simulink model "gm_Encoder_Zynq_vnl"  (R2018a)
settings: Solver=ode3  StartTime=0.0  StopTime=SimulationsDauer  RelTol=1e-3  EnableMultiTasking=on
undefined symbols (not defined in the file or in its folder): DiscIntNeverNeededParam, f_ISR, IncPerTurn, n_max, OverSamplingFactor, OverSamplingFactorInverse, Periode, Phase_Delay_A, Phase_Delay_B, PolePair, T_mech, TestDrehzahl_rpm
libraries: simulink x18, hdlsllib x2, dspsigops x2, dspswit3 x2, powerlib_meascontrol x2, hdlmdlgenlib x1, simulink_extras x1, powerlib x1
(part 1 of 3)
settings Model: Creator=Wendel_ELSYS  LastModifiedBy=Wendel
settings DataIOCC: LimitDataPoints=on  SaveFormat=Array
settings OptimizationCC: BlockReduction=off  ConditionallyExecuteInputs=off  DefaultParameterBehavior=Inlined  LifeSpan=inf
settings DebuggingCC: AlgebraicLoopMsg=error  InheritedTsInSrcMsg=none  ParameterOverflowMsg=none  SFUnexpectedBacktrackingDiag=warning  SFNoUnconditionalDefaultTransitionDiag=warning  SFExecutionAtInitializationDiag=none
settings HardwareCC: ProdBitPerPointer=32  ProdBitPerSizeT=32  ProdBitPerPtrDiffT=32  ProdLargestAtomicFloat=None  ProdIntDivRoundTo=Undefined  ProdEndianess=Unspecified  ProdWordSize=32  ProdHWDeviceType=ASIC/FPGA->ASIC/FPGA  ProdEqTarget=off
settings ModelReferenceCC: PropagateSignalLabelsOutOfModel=off
settings CodeAppCC: StateflowObjectComments=on
settings GRTTargetCC: TargetLangStandard=C89/C90 (ANSI)  GeneratePreprocessorConditionals=Disable all
settings ConfigComp: CovMetricSettings=dw  CovHtmlReporting=on  CovSaveCumulativeToWorkspaceVar=on  CovSaveSingleToWorkspaceVar=on  CovExternalEMLEnable=off
settings SimscapeCC: SimscapeNormalizeSystem=off

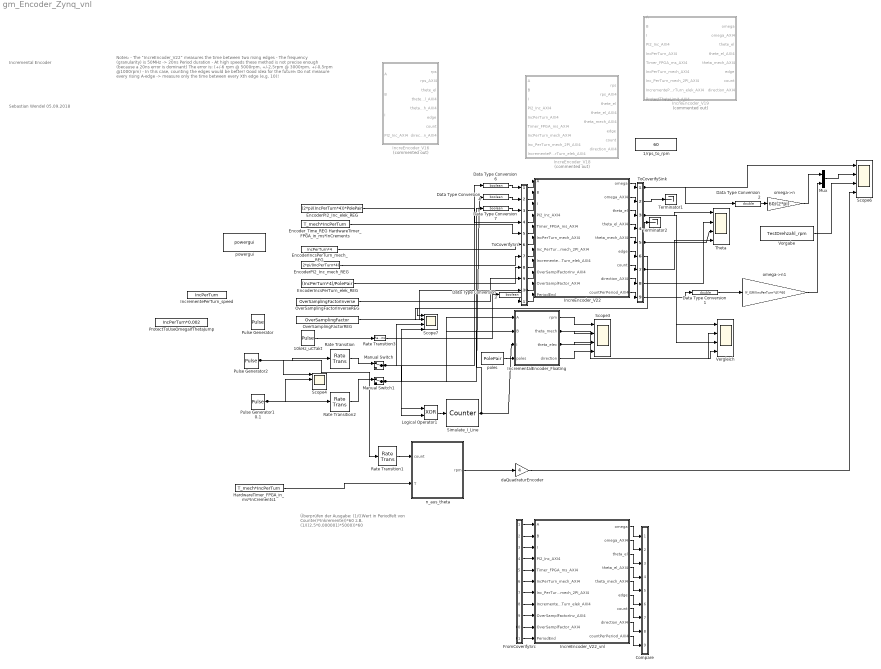
== system gm_Encoder_Zynq_vnl ==
  note: Überprüfen der Ausgabe:
      | (1/((Wert in Periodfelt von Counter)*Inkremente))*60
      | z.B. (1/((2.5*0.000001)*5000))*60
  note: Sebastian Wendel
      | 05.09.2018
  note: Notes:
      | - The "IncreEncoder_V22" measures the time between two rising edges
      | - The frequency (granularity) is 50MHz -> 20ns Period duration
      | - At high speeds these method is not precise enough (because a 20ns error is dominant)
      | The error is: (+/-6 rpm @ 5000rpm, +/-2,5rpm @ 3000rpm, +/-0,5rpm @1000rpm)
      | - In this case, counting the edges would be better!
      |
      | Good idea for the future: Do not measure every rising A-edge
      | -> measure only the time between every Xth edge (e.g. 10)!
  note: Incremental Encoder
  1/rps_to_rpm : Constant  Value=60  OutDataTypeStr=double  SampleTime=T_mech
  10kHz_uCTakt : DiscretePulseGenerator  PulseType=Time based  Period=0.000100  PulseWidth=0.0002  SampleTime=T_mech  VectorParams1D=off
  Compare : Subsystem
      mask Display: disp('')
  Data Type Conversion1 : DataTypeConversion  OutDataTypeStr=double
  Data Type Conversion2 : DataTypeConversion  OutDataTypeStr=double
  Data Type Conversion{3..4,6..7} (4 alike) : DataTypeConversion  OutDataTypeStr=boolean
  "EncoderIncsPerTurn_elek_REG " : Constant  Value=(IncPerTurn*4)/PolePair  OutDataTypeStr=fixdt(0,16,0)  SampleTime=T_mech
  EncoderIncsPerTurn_mech_REG : Constant  Value=IncPerTurn*4  OutDataTypeStr=fixdt(0,16,0)  SampleTime=T_mech
  EncoderPI2_Inc_elek_REG : Constant  Value=(2*pi/(IncPerTurn*4))*PolePair  OutDataTypeStr=fixdt(0,24,24)  SampleTime=T_mech
  EncoderPI2_Inc_mech_REG : Constant  Value=2*pi/(IncPerTurn*4)  OutDataTypeStr=fixdt(0,24,24)  SampleTime=T_mech
  Encoder_Time_REG HardwareTimer_FPGA_in_ms*InCrements : Constant  Value=T_mech*IncPerTurn  OutDataTypeStr=fixdt(0,32,26)  SampleTime=T_mech
  FromCoverifySrc : Subsystem
      mask Display: disp('')
  HardwareTimer_FPGA_in_ms*InCrements1 : Constant  Value=T_mech*IncPerTurn  OutDataTypeStr=double  SampleTime=T_mech
  IncreEncoder_V16 : Subsystem  Commented=on  TreatAsAtomicUnit=on
  IncreEncoder_V18 : Subsystem  Commented=on  TreatAsAtomicUnit=on
  IncreEncoder_V19 : Subsystem  Commented=on  TreatAsAtomicUnit=on
  IncreEncoder_V22 : Subsystem  TreatAsAtomicUnit=on
  IncreEncoder_V22_vnl : Subsystem  TreatAsAtomicUnit=on
  IncrementalEncoder_Floating : Subsystem
  IncrementePerTurn_speed : Constant  Value=IncPerTurn  OutDataTypeStr=fixdt(0,16,0)  SampleTime=T_mech
  Logical Operator1 : Logic  Operator=XOR  AllPortsSameDT=off  OutDataTypeStr=boolean
  Manual Switch : ManualSwitch
  Manual Switch1 : ManualSwitch
  Mux : Mux  Inputs=2
  OverSamplingFactorInverseREG : Constant  Value=OverSamplingFactorInverse  OutDataTypeStr=fixdt(0,16,15)  SampleTime=T_mech
  OverSamplingFactorREG : Constant  Value=OverSamplingFactor  OutDataTypeStr=fixdt(0,16,0)  SampleTime=T_mech
  ProtectToUseOmegaIfThetaJump : Constant  Value=IncPerTurn*0.002  OutDataTypeStr=uint16  SampleTime=T_mech
  Pulse Generator : DiscretePulseGenerator  PulseType=Time based  Period=0.01  PulseWidth=50  PhaseDelay=0.00000125  SampleTime=T_mech  VectorParams1D=off
  Pulse Generator1 0.1 : DiscretePulseGenerator  PulseType=Time based  Period=Periode  PulseWidth=50  PhaseDelay=Phase_Delay_B  SampleTime=T_mech  VectorParams1D=off
  Pulse Generator2 : DiscretePulseGenerator  PulseType=Time based  Period=Periode  PulseWidth=50  PhaseDelay=Phase_Delay_A  SampleTime=T_mech  VectorParams1D=off
  Rate Transition{,1..3} (4 alike) : RateTransition  Deterministic=off  OutPortSampleTime=T_mech
  Scope{3..4,6..7} (4 alike) : Scope  NumInputPorts=4
  Simulate_I_Line : dspswit3/Counter  Direction=Up  CountEvent=Either edge  CounterSize=User defined  MaxCount=IncPerTurn*4  InitialCount=0  Output=Hit  HitValue=IncPerTurn*4  ResetInput=off  SamplesPerFrame=1  Ts=1  CntDtype=double  HitDtype=Boolean
  Terminator1 : Terminator
  Terminator2 : Terminator
  Theta : Scope  NumInputPorts=4
  ToCoverifySink : Subsystem
      mask Display: disp('')
  ToCoverifySrc : Subsystem
      mask Display: disp('')
  Vergleich : Scope  NumInputPorts=4
  Vorgabe : Constant  Value=TestDrehzahl_rpm
  "daQuadraturEncoder " : Gain  Gain=4
  n_aus_theta : Subsystem  TreatAsAtomicUnit=on
  omega->n : Gain  Gain=60/(2*pi)  OutDataTypeStr=double
  omega->n1 : Gain  Gain=(f_ISR/(IncPerTurn*4))*60  OutDataTypeStr=double
  poles : Constant  Value=PolePair  OutDataTypeStr=uint8  SampleTime=-1
  powergui : powerlib/powergui  Priority=1  SimulationMode=Discrete  SampleTime=T_mech  frequency=60  Iterations=50  frequencyindice=0  Pbase=100e6  ErrMax=1e-4  UnitsV=kV  UnitsW=MW  buscounter=0  FunctionMessages=off  echomessages=off  EnableUseOfTLC=off  CurrentSourceSwitches=off  DisableSnubberDevices=off  DisableRonSwitches=off  DisableVfSwitches=off  DisplayEquations=off  SolverType=Tustin  Interpol=off  ExternalGateDelay=off  methode=off  Ts=0  x0status=blocks  SPID=off  SwTol=0  HookPort=off  RestoreLinks=warning  ResistiveCurrentMeasurement=off  Frange=[0:2:500]  Ylog=off  Xlog=on  ShowGrid=off  save=off  variable=ZData  structure=0  ZoomFFT=on  StartTime=0.0  cycles=1  DisplayStyle=1  fundamental=60  FreqAxis=off  MaxFrequency=1000  frequencyindicesteady=1  RmsSteady=1  display=off
  wires:
  Pulse Generator1 0.1/1 -> Scope4/2, Rate Transition2/1
  Manual Switch1/1 -> Logical Operator1/2, Scope7/4, IncrementalEncoder_Floating/2(B), Data Type Conversion4/1
  Simulate_I_Line/1 -> IncrementalEncoder_Floating/3(I), Data Type Conversion7/1
  Logical Operator1/1 -> Simulate_I_Line/1
  Manual Switch/1 -> Scope7/3, Data Type Conversion6/1, IncrementalEncoder_Floating/1(A), Logical Operator1/1
  IncrementalEncoder_Floating/1(rpm) -> Scope3/1
  IncrementalEncoder_Floating/2(theta_mech) -> Vergleich/4, Scope3/2
  IncrementalEncoder_Floating/3(theta_elec) -> Vergleich/2, Scope3/3
  IncrementalEncoder_Floating/4(direction) -> Scope3/4
  poles/1 -> IncrementalEncoder_Floating/4(poles)
  omega->n/1 -> Mux/1
  Data Type Conversion2/1 -> omega->n/1
  HardwareTimer_FPGA_in_ms*InCrements1/1 -> n_aus_theta/2(T)
  Rate Transition1/1 -> n_aus_theta/1(count)
  n_aus_theta/1(rpm) -> "daQuadraturEncoder "/1
  Pulse Generator2/1 -> Rate Transition/1, Scope4/1, Rate Transition1/1
  "daQuadraturEncoder "/1 -> Scope6/4
  Vorgabe/1 -> Scope6/3
  Rate Transition2/1 -> Manual Switch1/1
  Rate Transition/1 -> Manual Switch/1
  10kHz_uCTakt/1 -> Rate Transition3/1
  Rate Transition3/1 -> Data Type Conversion3/1
  Data Type Conversion1/1 -> omega->n1/1
  Mux/1 -> Scope6/2
  omega->n1/1 -> Mux/2
  ToCoverifySrc/1(out1) -> IncreEncoder_V22/1(A)
  ToCoverifySrc/2(out2) -> IncreEncoder_V22/2(B)
  ToCoverifySrc/3(out3) -> IncreEncoder_V22/3(I)
  ToCoverifySrc/4(out4) -> IncreEncoder_V22/4(PI2_Inc_AXI4)
  ToCoverifySrc/5(out5) -> IncreEncoder_V22/5(Timer_FPGA_ms_AXI4)
  ToCoverifySrc/6(out6) -> IncreEncoder_V22/6(IncPerTurn_mech_AXI4)
  ToCoverifySrc/7(out7) -> IncreEncoder_V22/7(Inc_PerTurn_mech_2PI_AXI4)
  ToCoverifySrc/8(out8) -> IncreEncoder_V22/8(IncrementePerTurn_elek_AXI4)
  ToCoverifySrc/9(out9) -> IncreEncoder_V22/9(OverSamplFactorInv_AXI4)
  ToCoverifySrc/10(out10) -> IncreEncoder_V22/10(OverSamplFactor_AXI4)
  ToCoverifySrc/11(out11) -> IncreEncoder_V22/11(PeriodEnd)
  IncreEncoder_V22/1(omega) -> ToCoverifySink/1(in1)
  IncreEncoder_V22/2(omega_AXI4) -> ToCoverifySink/2(in2)
  IncreEncoder_V22/3(theta_el) -> ToCoverifySink/3(in3)
  IncreEncoder_V22/4(theta_el_AXI4) -> ToCoverifySink/4(in4)
  IncreEncoder_V22/5(theta_mech_AXI4) -> ToCoverifySink/5(in5)
  IncreEncoder_V22/6(edge) -> ToCoverifySink/6(in6)
  IncreEncoder_V22/7(count) -> ToCoverifySink/7(in7)
  IncreEncoder_V22/8(direction_AXI4) -> ToCoverifySink/8(in8)
  IncreEncoder_V22/9(countPerPeriod_AXI4) -> ToCoverifySink/9(in9)
  Data Type Conversion6/1 -> ToCoverifySrc/1(in1)
  Data Type Conversion4/1 -> ToCoverifySrc/2(in2)
  Data Type Conversion7/1 -> ToCoverifySrc/3(in3)
  EncoderPI2_Inc_elek_REG/1 -> ToCoverifySrc/4(in4)
  Encoder_Time_REG HardwareTimer_FPGA_in_ms*InCrements/1 -> ToCoverifySrc/5(in5)
  EncoderIncsPerTurn_mech_REG/1 -> ToCoverifySrc/6(in6)
  EncoderPI2_Inc_mech_REG/1 -> ToCoverifySrc/7(in7)
  "EncoderIncsPerTurn_elek_REG "/1 -> ToCoverifySrc/8(in8)
  OverSamplingFactorInverseREG/1 -> ToCoverifySrc/9(in9)
  OverSamplingFactorREG/1 -> ToCoverifySrc/10(in10)
  Data Type Conversion3/1 -> ToCoverifySrc/11(in11)
  ToCoverifySink/1(out1) -> Data Type Conversion2/1, Scope6/1
  ToCoverifySink/2(out2) -> Terminator1/1
  ToCoverifySink/3(out3) -> Vergleich/1, Theta/1
  ToCoverifySink/4(out4) -> Terminator2/1
  ToCoverifySink/5(out5) -> Theta/3, Vergleich/3
  ToCoverifySink/6(out6) -> Scope7/1
  ToCoverifySink/7(out7) -> Scope7/2, Theta/4
  ToCoverifySink/8(out8) -> Theta/2
  ToCoverifySink/9(out9) -> Data Type Conversion1/1
  FromCoverifySrc/1(out1) -> IncreEncoder_V22_vnl/1(A)
  FromCoverifySrc/2(out2) -> IncreEncoder_V22_vnl/2(B)
  FromCoverifySrc/3(out3) -> IncreEncoder_V22_vnl/3(I)
  FromCoverifySrc/4(out4) -> IncreEncoder_V22_vnl/4(PI2_Inc_AXI4)
  FromCoverifySrc/5(out5) -> IncreEncoder_V22_vnl/5(Timer_FPGA_ms_AXI4)
  FromCoverifySrc/6(out6) -> IncreEncoder_V22_vnl/6(IncPerTurn_mech_AXI4)
  FromCoverifySrc/7(out7) -> IncreEncoder_V22_vnl/7(Inc_PerTurn_mech_2PI_AXI4)
  FromCoverifySrc/8(out8) -> IncreEncoder_V22_vnl/8(IncrementePerTurn_elek_AXI4)
  FromCoverifySrc/9(out9) -> IncreEncoder_V22_vnl/9(OverSamplFactorInv_AXI4)
  FromCoverifySrc/10(out10) -> IncreEncoder_V22_vnl/10(OverSamplFactor_AXI4)
  FromCoverifySrc/11(out11) -> IncreEncoder_V22_vnl/11(PeriodEnd)
  IncreEncoder_V22_vnl/1(omega) -> Compare/1(in1)
  IncreEncoder_V22_vnl/2(omega_AXI4) -> Compare/2(in2)
  IncreEncoder_V22_vnl/3(theta_el) -> Compare/3(in3)
  IncreEncoder_V22_vnl/4(theta_el_AXI4) -> Compare/4(in4)
  IncreEncoder_V22_vnl/5(theta_mech_AXI4) -> Compare/5(in5)
  IncreEncoder_V22_vnl/6(edge) -> Compare/6(in6)
  IncreEncoder_V22_vnl/7(count) -> Compare/7(in7)
  IncreEncoder_V22_vnl/8(direction_AXI4) -> Compare/8(in8)
  IncreEncoder_V22_vnl/9(countPerPeriod_AXI4) -> Compare/9(in9)

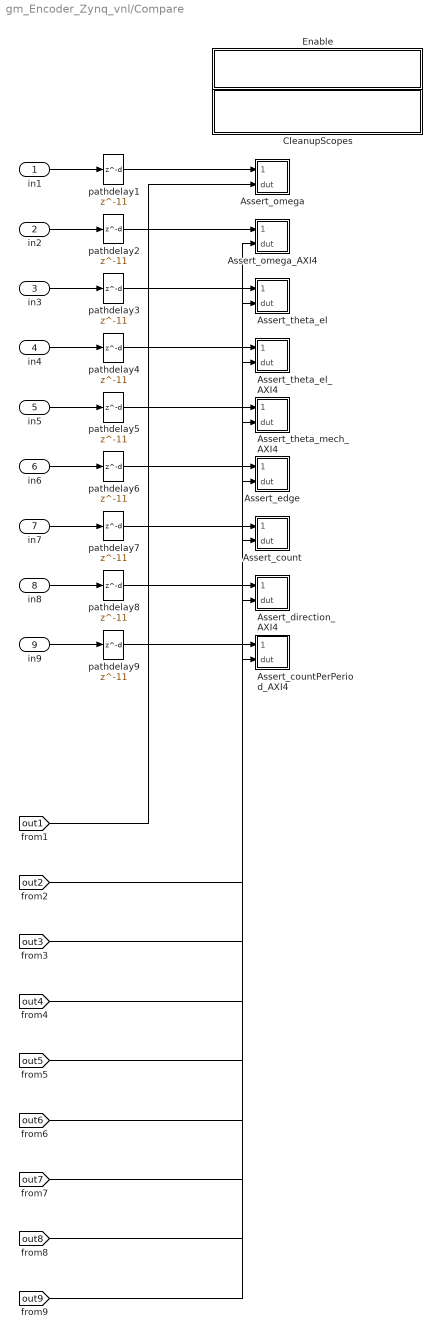
== system gm_Encoder_Zynq_vnl/Compare ==
  in1 : Inport
  in2 : Inport  Port=2
  in3 : Inport  Port=3
  in4 : Inport  Port=4
  in5 : Inport  Port=5
  in6 : Inport  Port=6
  in7 : Inport  Port=7
  in8 : Inport  Port=8
  in9 : Inport  Port=9
  Assert_count : Subsystem
  Assert_countPerPeriod_AXI4 : Subsystem
  Assert_direction_AXI4 : Subsystem
  Assert_edge : Subsystem
  Assert_omega : Subsystem
  Assert_omega_AXI4 : Subsystem
  Assert_theta_el : Subsystem
  Assert_theta_el_AXI4 : Subsystem
  Assert_theta_mech_AXI4 : Subsystem
  CleanupScopes : Subsystem
      settings: OpenFcn=|
      | blkName = gcb; %self block
      | idx = regexp(blkName, '/CleanupScopes$', 'once');
      | blkParent = blkName(1:idx-1);
      | blks=find_system(blkParent, 'LookUnderMasks', 'all','blocktype', 'Scope');
      | for itr = 1:length(blks)
      | 	 hScopeCfg = get_param(blks{itr},'ScopeConfiguration');
      | 	 hScopeCfg.Visible = ~ hScopeCfg.Visible;
      | end
      | drawnow;
      mask Display: fprintf(message('hdlcoder:cosim:vnl_dblclick').getString());
  Enable : Subsystem
      settings: OpenFcn=|
      | blkName = gcb;
      | idx = regexp(blkName, '/Enable$', 'once');
      | blkParent = blkName(1:idx-1);
      | blks=find_system(blkParent, 'LookUnderMasks', 'all','blocktype', 'Assertion');
      | e = get_param(blks{1}, 'Enabled');
      | if strcmp(e, 'on'), f= 'off';, else, f = 'on';, end
      | for ii=1:length(blks), set_param(blks{ii}, 'Enabled', f);, end
      | set_param(gcb, 'MaskDisplay',['fprintf(message(''hdlcoder:cosim:vnl_dblclick_assertions'',','''',upper(e),'''',').getString())']);
      mask Display: fprintf(message('hdlcoder:cosim:vnl_dblclick_assertions','OFF').getString());
  pathdelay{1..9} (9 alike) : Delay  DelayLength=11
  wires:
  in1/1 -> pathdelay1/1
  pathdelay1/1 -> Assert_omega/1(cosim)
  [out1] -> Assert_omega/2(dut)
  in2/1 -> pathdelay2/1
  pathdelay2/1 -> Assert_omega_AXI4/1(cosim)
  [out2] -> Assert_omega_AXI4/2(dut)
  in3/1 -> pathdelay3/1
  pathdelay3/1 -> Assert_theta_el/1(cosim)
  [out3] -> Assert_theta_el/2(dut)
  in4/1 -> pathdelay4/1
  pathdelay4/1 -> Assert_theta_el_AXI4/1(cosim)
  [out4] -> Assert_theta_el_AXI4/2(dut)
  in5/1 -> pathdelay5/1
  pathdelay5/1 -> Assert_theta_mech_AXI4/1(cosim)
  [out5] -> Assert_theta_mech_AXI4/2(dut)
  in6/1 -> pathdelay6/1
  pathdelay6/1 -> Assert_edge/1(cosim)
  [out6] -> Assert_edge/2(dut)
  in7/1 -> pathdelay7/1
  pathdelay7/1 -> Assert_count/1(cosim)
  [out7] -> Assert_count/2(dut)
  in8/1 -> pathdelay8/1
  pathdelay8/1 -> Assert_direction_AXI4/1(cosim)
  [out8] -> Assert_direction_AXI4/2(dut)
  in9/1 -> pathdelay9/1
  pathdelay9/1 -> Assert_countPerPeriod_AXI4/1(cosim)
  [out9] -> Assert_countPerPeriod_AXI4/2(dut)

== system gm_Encoder_Zynq_vnl/FromCoverifySrc ==
  out1 : Outport
  out2 : Outport  Port=2
  out3 : Outport  Port=3
  out4 : Outport  Port=4
  out5 : Outport  Port=5
  out6 : Outport  Port=6
  out7 : Outport  Port=7
  out8 : Outport  Port=8
  out9 : Outport  Port=9
  out10 : Outport  Port=10
  out11 : Outport  Port=11
  wires:
  [in1] -> out1/1
  [in2] -> out2/1
  [in3] -> out3/1
  [in4] -> out4/1
  [in5] -> out5/1
  [in6] -> out6/1
  [in7] -> out7/1
  [in8] -> out8/1
  [in9] -> out9/1
  [in10] -> out10/1
  [in11] -> out11/1

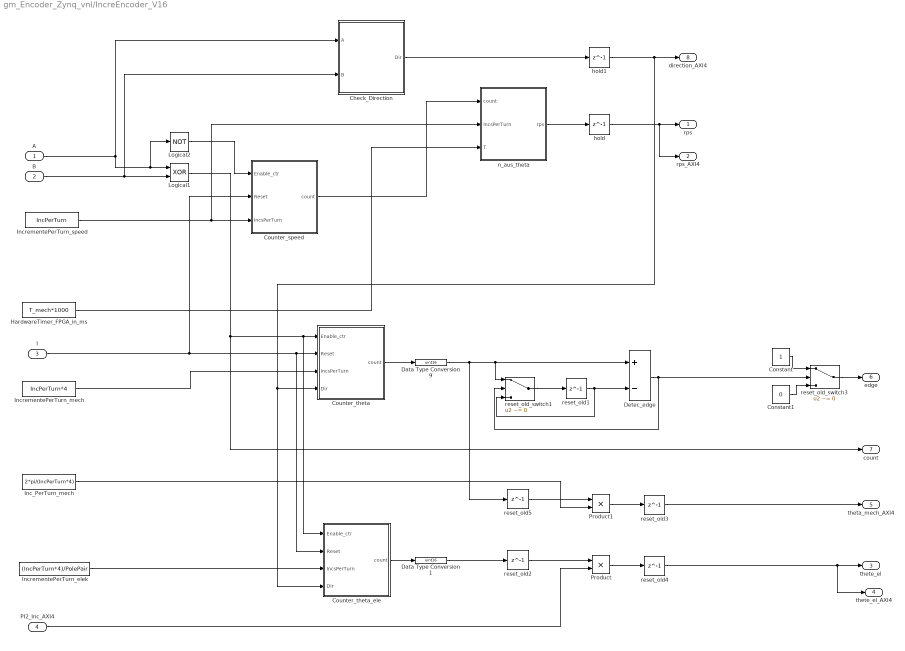
== system gm_Encoder_Zynq_vnl/IncreEncoder_V16 ==
  A : Inport
  B : Inport  Port=2
  I : Inport  Port=3
  PI2_Inc_AXI4 : Inport  Port=4
  Check_Direction : Subsystem  TreatAsAtomicUnit=on
  Constant : Constant  OutDataTypeStr=boolean  SampleTime=-1
  Constant1 : Constant  Value=0  OutDataTypeStr=boolean  SampleTime=-1
  Counter_speed : Subsystem  TreatAsAtomicUnit=on
  Counter_theta : Subsystem  TreatAsAtomicUnit=on
  Counter_theta_ele : Subsystem  TreatAsAtomicUnit=on
  Data Type Conversion1 : DataTypeConversion  OutDataTypeStr=uint16
  Data Type Conversion9 : DataTypeConversion  OutDataTypeStr=uint16
  Detec_edge : Sum  Inputs=+-  AccumDataTypeStr=uint8  OutDataTypeStr=uint8
  HardwareTimer_FPGA_in_ms : Constant  Value=T_mech*1000  OutDataTypeStr=fixdt(0,30,24)  SampleTime=T_mech
  Inc_PerTurn_mech : Constant  Value=2*pi/(IncPerTurn*4)  OutDataTypeStr=fixdt(0,24,24)  SampleTime=T_mech
  IncrementePerTurn_elek : Constant  Value=(IncPerTurn*4)/PolePair  OutDataTypeStr=fixdt(0,16,0)  SampleTime=T_mech
  IncrementePerTurn_mech : Constant  Value=IncPerTurn*4  OutDataTypeStr=fixdt(0,16,0)  SampleTime=T_mech
  IncrementePerTurn_speed : Constant  Value=IncPerTurn  OutDataTypeStr=fixdt(0,16,0)  SampleTime=T_mech
  Logical1 : Logic  Operator=XOR  AllPortsSameDT=off  OutDataTypeStr=boolean
  Logical2 : Logic  Operator=NOT  AllPortsSameDT=off  OutDataTypeStr=boolean
  Product : Product  OutDataTypeStr=fixdt(0,24,20)
  Product1 : Product  OutDataTypeStr=fixdt(0,24,20)
  hold : Delay  DelayLength=1
  hold1 : Delay  DelayLength=1
  n_aus_theta : Subsystem  TreatAsAtomicUnit=on
  reset_old{1..5} (5 alike) : Delay  DelayLength=1
  reset_old_switch1 : Switch  Criteria=u2 ~= 0
  reset_old_switch3 : Switch  Criteria=u2 ~= 0
  rps : Outport
  rps_AXI4 : Outport  Port=2
  thete_el : Outport  Port=3
  thete_el_AXI4 : Outport  Port=4
  theta_mech_AXI4 : Outport  Port=5
  edge : Outport  Port=6
  count : Outport  Port=7
  direction_AXI4 : Outport  Port=8
  wires:
  A/1 -> Check_Direction/1(A), Logical2/1, Logical1/1
  B/1 -> Check_Direction/2(B), Logical1/2
  I/1 -> Counter_speed/2(Reset), Counter_theta_ele/2(Reset), Counter_theta/2(Reset)
  IncrementePerTurn_speed/1 -> Counter_speed/3(IncsPerTurn), n_aus_theta/2(IncsPerTurn)
  Check_Direction/1(Dir) -> hold1/1
  hold/1 -> rps_AXI4/1, rps/1
  hold1/1 -> Counter_theta_ele/4(Dir), Counter_theta/4(Dir), direction_AXI4/1
  Counter_theta/1(count) -> Data Type Conversion9/1
  reset_old_switch1/1 -> reset_old1/1
  reset_old1/1 -> reset_old_switch1/3, Detec_edge/2
  reset_old3/1 -> theta_mech_AXI4/1
  Product1/1 -> reset_old3/1
  Inc_PerTurn_mech/1 -> Product1/2
  Product/1 -> reset_old4/1
  Constant/1 -> reset_old_switch3/1
  reset_old_switch3/1 -> edge/1
  Constant1/1 -> reset_old_switch3/3
  Detec_edge/1 -> reset_old_switch3/2, reset_old_switch1/2
  Logical1/1 -> count/1, Counter_theta_ele/1(Enable_ctr), Counter_theta/1(Enable_ctr)
  Counter_speed/1(count) -> n_aus_theta/1(count)
  IncrementePerTurn_mech/1 -> Counter_theta/3(IncsPerTurn)
  n_aus_theta/1(rps) -> hold/1
  Data Type Conversion9/1 -> reset_old5/1, Detec_edge/1, reset_old_switch1/1
  IncrementePerTurn_elek/1 -> Counter_theta_ele/3(IncsPerTurn)
  PI2_Inc_AXI4/1 -> Product/2
  Counter_theta_ele/1(count) -> Data Type Conversion1/1
  reset_old4/1 -> thete_el_AXI4/1, thete_el/1
  Data Type Conversion1/1 -> reset_old2/1
  reset_old2/1 -> Product/1
  reset_old5/1 -> Product1/1
  Logical2/1 -> Counter_speed/1(Enable_ctr)
  HardwareTimer_FPGA_in_ms/1 -> n_aus_theta/3(T)

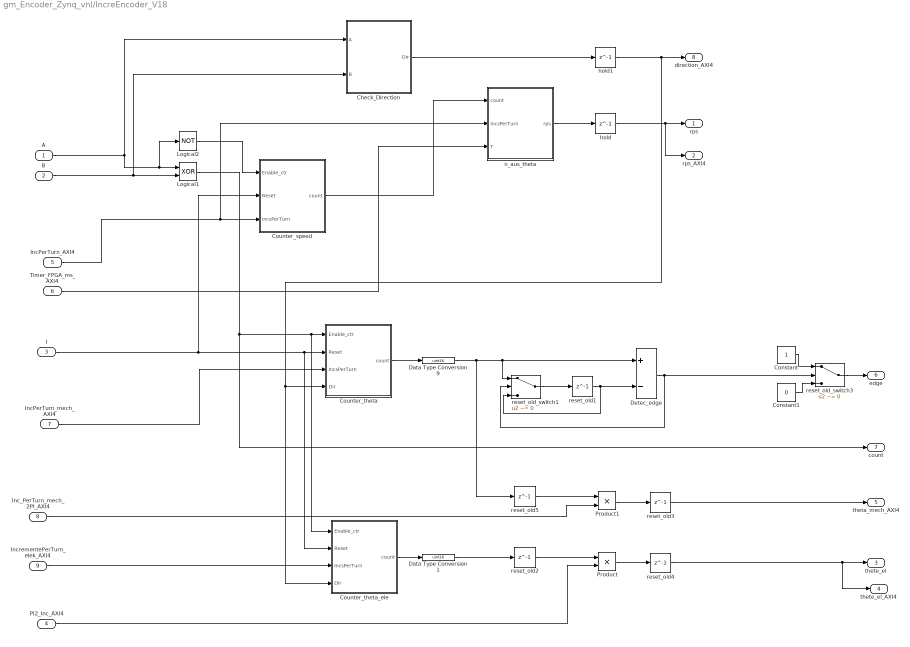
== system gm_Encoder_Zynq_vnl/IncreEncoder_V18 ==
  A : Inport
  B : Inport  Port=2
  I : Inport  Port=3
  PI2_Inc_AXI4 : Inport  Port=4
  IncPerTurn_AXI4 : Inport  Port=5
  Timer_FPGA_ms_AXI4 : Inport  Port=6
  IncPerTurn_mech_AXI4 : Inport  Port=7
  Inc_PerTurn_mech_2PI_AXI4 : Inport  Port=8
  IncrementePerTurn_elek_AXI4 : Inport  Port=9
  Check_Direction : Subsystem  TreatAsAtomicUnit=on
  Constant : Constant  OutDataTypeStr=boolean  SampleTime=-1
  Constant1 : Constant  Value=0  OutDataTypeStr=boolean  SampleTime=-1
  Counter_speed : Subsystem  TreatAsAtomicUnit=on
  Counter_theta : Subsystem  TreatAsAtomicUnit=on
  Counter_theta_ele : Subsystem  TreatAsAtomicUnit=on
  Data Type Conversion1 : DataTypeConversion  OutDataTypeStr=uint16
  Data Type Conversion9 : DataTypeConversion  OutDataTypeStr=uint16
  Detec_edge : Sum  Inputs=+-  AccumDataTypeStr=uint8  OutDataTypeStr=uint8
  Logical1 : Logic  Operator=XOR  AllPortsSameDT=off  OutDataTypeStr=boolean
  Logical2 : Logic  Operator=NOT  AllPortsSameDT=off  OutDataTypeStr=boolean
  Product : Product  OutDataTypeStr=fixdt(1,24,20)
  Product1 : Product  OutDataTypeStr=fixdt(1,24,20)
  hold : Delay  DelayLength=1
  hold1 : Delay  DelayLength=1
  n_aus_theta : Subsystem  TreatAsAtomicUnit=on
  reset_old{1..5} (5 alike) : Delay  DelayLength=1
  reset_old_switch1 : Switch  Criteria=u2 ~= 0
  reset_old_switch3 : Switch  Criteria=u2 ~= 0
  rps : Outport
  rps_AXI4 : Outport  Port=2
  thete_el : Outport  Port=3
  thete_el_AXI4 : Outport  Port=4
  theta_mech_AXI4 : Outport  Port=5
  edge : Outport  Port=6
  count : Outport  Port=7
  direction_AXI4 : Outport  Port=8
  wires:
  A/1 -> Check_Direction/1(A), Logical2/1, Logical1/1
  B/1 -> Check_Direction/2(B), Logical1/2
  I/1 -> Counter_speed/2(Reset), Counter_theta_ele/2(Reset), Counter_theta/2(Reset)
  IncPerTurn_AXI4/1 -> Counter_speed/3(IncsPerTurn), n_aus_theta/2(IncsPerTurn)
  Check_Direction/1(Dir) -> hold1/1
  hold/1 -> rps_AXI4/1, rps/1
  hold1/1 -> Counter_theta_ele/4(Dir), Counter_theta/4(Dir), direction_AXI4/1
  Counter_theta/1(count) -> Data Type Conversion9/1
  reset_old_switch1/1 -> reset_old1/1
  reset_old1/1 -> reset_old_switch1/3, Detec_edge/2
  reset_old3/1 -> theta_mech_AXI4/1
  Product1/1 -> reset_old3/1
  Inc_PerTurn_mech_2PI_AXI4/1 -> Product1/2
  Product/1 -> reset_old4/1
  Constant/1 -> reset_old_switch3/1
  reset_old_switch3/1 -> edge/1
  Constant1/1 -> reset_old_switch3/3
  Detec_edge/1 -> reset_old_switch3/2, reset_old_switch1/2
  Logical1/1 -> count/1, Counter_theta_ele/1(Enable_ctr), Counter_theta/1(Enable_ctr)
  Counter_speed/1(count) -> n_aus_theta/1(count)
  IncPerTurn_mech_AXI4/1 -> Counter_theta/3(IncsPerTurn)
  n_aus_theta/1(rps) -> hold/1
  Data Type Conversion9/1 -> reset_old5/1, Detec_edge/1, reset_old_switch1/1
  IncrementePerTurn_elek_AXI4/1 -> Counter_theta_ele/3(IncsPerTurn)
  PI2_Inc_AXI4/1 -> Product/2
  Counter_theta_ele/1(count) -> Data Type Conversion1/1
  reset_old4/1 -> thete_el_AXI4/1, thete_el/1
  Data Type Conversion1/1 -> reset_old2/1
  reset_old2/1 -> Product/1
  reset_old5/1 -> Product1/1
  Logical2/1 -> Counter_speed/1(Enable_ctr)
  Timer_FPGA_ms_AXI4/1 -> n_aus_theta/3(T)

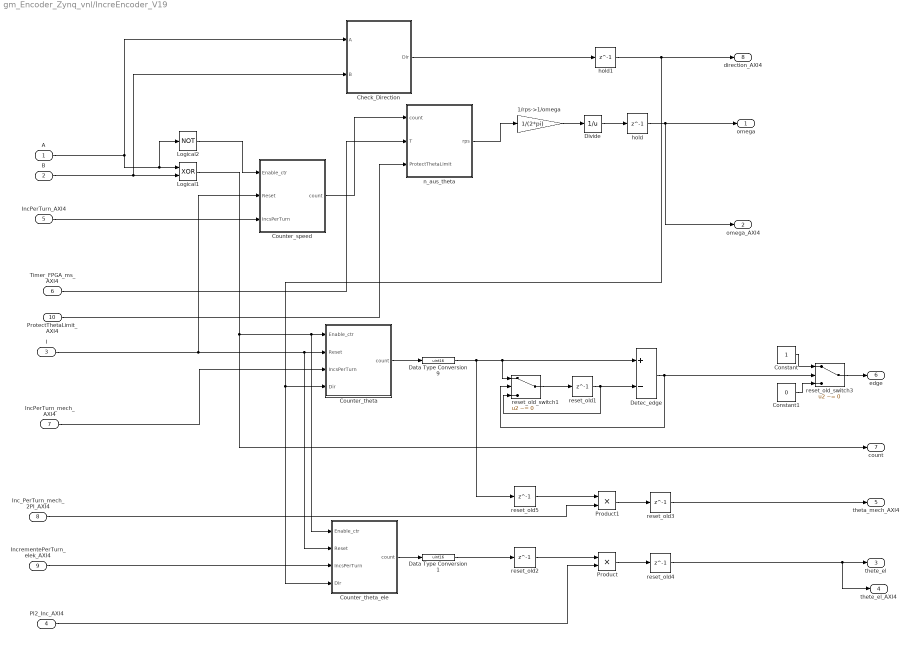
== system gm_Encoder_Zynq_vnl/IncreEncoder_V19 ==
  A : Inport
  B : Inport  Port=2
  I : Inport  Port=3
  PI2_Inc_AXI4 : Inport  Port=4
  IncPerTurn_AXI4 : Inport  Port=5
  Timer_FPGA_ms_AXI4 : Inport  Port=6
  IncPerTurn_mech_AXI4 : Inport  Port=7
  Inc_PerTurn_mech_2PI_AXI4 : Inport  Port=8
  IncrementePerTurn_elek_AXI4 : Inport  Port=9
  ProtectThetaLimit_AXI4 : Inport  Port=10
  1/rps->1/omega : Gain  Gain=1/(2*pi)  OutDataTypeStr=fixdt(1,24,18)
  Check_Direction : Subsystem  TreatAsAtomicUnit=on
  Constant : Constant  OutDataTypeStr=boolean  SampleTime=-1
  Constant1 : Constant  Value=0  OutDataTypeStr=boolean  SampleTime=-1
  Counter_speed : Subsystem  TreatAsAtomicUnit=on
  Counter_theta : Subsystem  TreatAsAtomicUnit=on
  Counter_theta_ele : Subsystem  TreatAsAtomicUnit=on
  Data Type Conversion1 : DataTypeConversion  OutDataTypeStr=uint16
  Data Type Conversion9 : DataTypeConversion  OutDataTypeStr=uint16
  Detec_edge : Sum  Inputs=+-  AccumDataTypeStr=uint8  OutDataTypeStr=uint8
  Divide : Math  Operator=reciprocal  OutDataTypeStr=fixdt(1,24,11)  RndMeth=Zero  SaturateOnIntegerOverflow=on
  Logical1 : Logic  Operator=XOR  AllPortsSameDT=off  OutDataTypeStr=boolean
  Logical2 : Logic  Operator=NOT  AllPortsSameDT=off  OutDataTypeStr=boolean
  Product : Product  OutDataTypeStr=fixdt(1,24,20)
  Product1 : Product  OutDataTypeStr=fixdt(1,24,20)
  hold : Delay  DelayLength=1
  hold1 : Delay  DelayLength=1
  n_aus_theta : Subsystem  TreatAsAtomicUnit=on
  reset_old{1..5} (5 alike) : Delay  DelayLength=1
  reset_old_switch1 : Switch  Criteria=u2 ~= 0
  reset_old_switch3 : Switch  Criteria=u2 ~= 0
  omega : Outport
  omega_AXI4 : Outport  Port=2
  thete_el : Outport  Port=3
  thete_el_AXI4 : Outport  Port=4
  theta_mech_AXI4 : Outport  Port=5
  edge : Outport  Port=6
  count : Outport  Port=7
  direction_AXI4 : Outport  Port=8
  wires:
  A/1 -> Check_Direction/1(A), Logical2/1, Logical1/1
  B/1 -> Check_Direction/2(B), Logical1/2
  I/1 -> Counter_speed/2(Reset), Counter_theta_ele/2(Reset), Counter_theta/2(Reset)
  IncPerTurn_AXI4/1 -> Counter_speed/3(IncsPerTurn)
  Check_Direction/1(Dir) -> hold1/1
  hold/1 -> omega_AXI4/1, omega/1
  hold1/1 -> Counter_theta_ele/4(Dir), Counter_theta/4(Dir), direction_AXI4/1
  Counter_theta/1(count) -> Data Type Conversion9/1
  reset_old_switch1/1 -> reset_old1/1
  reset_old1/1 -> reset_old_switch1/3, Detec_edge/2
  reset_old3/1 -> theta_mech_AXI4/1
  Product1/1 -> reset_old3/1
  Inc_PerTurn_mech_2PI_AXI4/1 -> Product1/2
  Product/1 -> reset_old4/1
  Constant/1 -> reset_old_switch3/1
  reset_old_switch3/1 -> edge/1
  Constant1/1 -> reset_old_switch3/3
  Detec_edge/1 -> reset_old_switch3/2, reset_old_switch1/2
  Logical1/1 -> count/1, Counter_theta_ele/1(Enable_ctr), Counter_theta/1(Enable_ctr)
  Counter_speed/1(count) -> n_aus_theta/1(count)
  IncPerTurn_mech_AXI4/1 -> Counter_theta/3(IncsPerTurn)
  n_aus_theta/1(rps) -> 1/rps->1/omega/1
  Data Type Conversion9/1 -> reset_old5/1, Detec_edge/1, reset_old_switch1/1
  IncrementePerTurn_elek_AXI4/1 -> Counter_theta_ele/3(IncsPerTurn)
  PI2_Inc_AXI4/1 -> Product/2
  Counter_theta_ele/1(count) -> Data Type Conversion1/1
  reset_old4/1 -> thete_el_AXI4/1, thete_el/1
  Data Type Conversion1/1 -> reset_old2/1
  reset_old2/1 -> Product/1
  reset_old5/1 -> Product1/1
  Logical2/1 -> Counter_speed/1(Enable_ctr)
  Timer_FPGA_ms_AXI4/1 -> n_aus_theta/2(T)
  Divide/1 -> hold/1
  1/rps->1/omega/1 -> Divide/1
  ProtectThetaLimit_AXI4/1 -> n_aus_theta/3(ProtectThetaLimit)

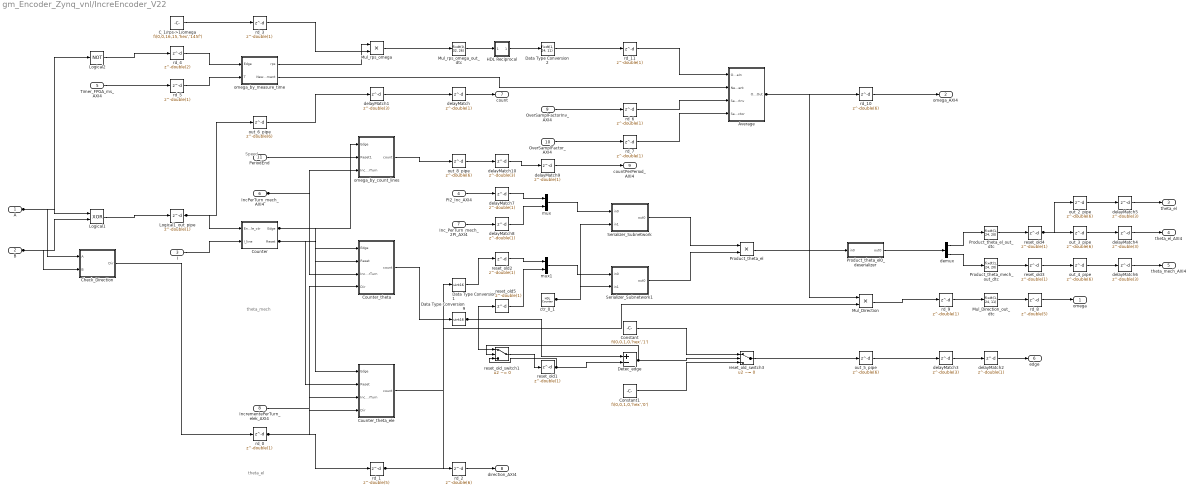
== system gm_Encoder_Zynq_vnl/IncreEncoder_V22 ==
  note: Speed
  note: theta_mech
  note: theta_el
  A : Inport  OutDataTypeStr=boolean  PortDimensions=1  SampleTime=2e-08
  B : Inport  Port=2  OutDataTypeStr=boolean  PortDimensions=1  SampleTime=2e-08
  I : Inport  Port=3  OutDataTypeStr=boolean  PortDimensions=1  SampleTime=2e-08
  PI2_Inc_AXI4 : Inport  Port=4  OutDataTypeStr=fixdt(0, 24, 24)  PortDimensions=1  SampleTime=2e-08
  Timer_FPGA_ms_AXI4 : Inport  Port=5  OutDataTypeStr=fixdt(0, 32, 26)  PortDimensions=1  SampleTime=2e-08
  IncPerTurn_mech_AXI4 : Inport  Port=6  OutDataTypeStr=uint16  PortDimensions=1  SampleTime=2e-08
  Inc_PerTurn_mech_2PI_AXI4 : Inport  Port=7  OutDataTypeStr=fixdt(0, 24, 24)  PortDimensions=1  SampleTime=2e-08
  IncrementePerTurn_elek_AXI4 : Inport  Port=8  OutDataTypeStr=uint16  PortDimensions=1  SampleTime=2e-08
  OverSamplFactorInv_AXI4 : Inport  Port=9  OutDataTypeStr=fixdt(0, 16, 15)  PortDimensions=1  SampleTime=2e-08
  OverSamplFactor_AXI4 : Inport  Port=10  OutDataTypeStr=uint16  PortDimensions=1  SampleTime=2e-08
  PeriodEnd : Inport  Port=11  OutDataTypeStr=boolean  PortDimensions=1  SampleTime=2e-08
  Average : Subsystem
  C_1/rps->1/omega : Constant  Value=fi(0,0,16,15,'hex','145f')  OutDataTypeStr=fixdt(0, 16, 15)  SampleTime=-1
  Check_Direction : Subsystem
  Constant : Constant  Value=fi(0,0,1,0,'hex','1')  OutDataTypeStr=boolean  SampleTime=-1
  Constant1 : Constant  Value=fi(0,0,1,0,'hex','0')  OutDataTypeStr=boolean  SampleTime=-1
  Counter : Subsystem
  Counter_theta : Subsystem
  Counter_theta_ele : Subsystem
  Data Type Conversion1 : DataTypeConversion  OutDataTypeStr=uint16  SampleTime=2e-08
  Data Type Conversion2 : DataTypeConversion  OutDataTypeStr=fixdt(1, 24, 11)  SampleTime=2e-08
  Data Type Conversion9 : DataTypeConversion  OutDataTypeStr=uint16  SampleTime=2e-08
  Detec_edge : Sum  Inputs=+-  AccumDataTypeStr=uint8  OutDataTypeStr=uint8  SampleTime=2e-08
  HDL Reciprocal : Subsystem
  Logical1 : Logic  Operator=XOR  AllPortsSameDT=off  OutDataTypeStr=boolean  SampleTime=2e-08
  Logical1_out_pipe : Delay  DelayLength=double(1)  InitialCondition=0  InputProcessing=Inherited  SampleTime=2e-08
  Logical2 : Logic  Operator=NOT  Inputs=1  AllPortsSameDT=off  OutDataTypeStr=boolean  SampleTime=2e-08
  Mul_Direction : Product  Inputs=**  OutDataTypeStr=fixdt(1, 28, 11)  SampleTime=2e-08
  Mul_Direction_out_dtc : DataTypeConversion  OutDataTypeStr=fixdt(1, 24, 11)  SampleTime=2e-08  SaturateOnIntegerOverflow=on  RndMeth=Zero
  Mul_rps_omega : Product  Inputs=**  OutDataTypeStr=fixdt(0, 48, 41)  SampleTime=2e-08
  Mul_rps_omega_out_dtc : DataTypeConversion  OutDataTypeStr=fixdt(0, 32, 26)  SampleTime=2e-08  SaturateOnIntegerOverflow=on  RndMeth=Zero
  Product_theta_el : Product  Inputs=**  OutDataTypeStr=fixdt(0, 40, 24)  SampleTime=1e-08
  Product_theta_el0_deserializer : Subsystem
  Product_theta_el_out_dtc : DataTypeConversion  OutDataTypeStr=fixdt(1, 24, 20)  SampleTime=2e-08
  Product_theta_mech_out_dtc : DataTypeConversion  OutDataTypeStr=fixdt(1, 24, 20)  SampleTime=2e-08
  Serializer_Subnetwork : Subsystem
  Serializer_Subnetwork1 : Subsystem
  ctr_0_1 : hdlsllib/Sources/HDL Counter  CountType=Count limited  CountInit=double(0)  CountStep=double(1)  CountMax=double(1)  CountFromType=Initial value  CountFrom=double(0)  CountResetPort=off  CountLoadPort=off  CountEnbPort=off  CountDirPort=off  CountDataType=Unsigned  CountWordLen=1  CountFracLen=0  CountSampTime=1e-08
      settings: SourceProductBaseCode=HD
  delayMatch{,2,7..9} (5 alike) : Delay  DelayLength=double(1)  InitialCondition=0  InputProcessing=Inherited  SampleTime=2e-08
  delayMatch{1,3..6,10} (6 alike) : Delay  DelayLength=double(3)  InitialCondition=0  InputProcessing=Inherited  SampleTime=2e-08
  demux : Demux  Outputs=2
  mux : Mux  Inputs=2
  mux1 : Mux  Inputs=2
  omega_by_count_lines : Subsystem
  omega_by_measure_time : Subsystem
  out_2_pipe : Delay  DelayLength=double(6)  InitialCondition=0  InputProcessing=Inherited  SampleTime=2e-08
  out_3_pipe : Delay  DelayLength=double(6)  InitialCondition=0  InputProcessing=Inherited  SampleTime=2e-08
  out_4_pipe : Delay  DelayLength=double(6)  InitialCondition=0  InputProcessing=Inherited  SampleTime=2e-08
  out_5_pipe : Delay  DelayLength=double(6)  InitialCondition=0  InputProcessing=Inherited  SampleTime=2e-08
  out_6_pipe : Delay  DelayLength=double(6)  InitialCondition=0  InputProcessing=Inherited  SampleTime=2e-08
  out_8_pipe : Delay  DelayLength=double(6)  InitialCondition=0  InputProcessing=Inherited  SampleTime=2e-08
  rd_{0,3,5..7,9,11} (7 alike) : Delay  DelayLength=double(1)  InitialCondition=0  InputProcessing=Inherited  SampleTime=2e-08
  rd_1 : Delay  DelayLength=double(5)  InitialCondition=0  InputProcessing=Inherited  SampleTime=2e-08
  rd_10 : Delay  DelayLength=double(6)  InitialCondition=0  InputProcessing=Inherited  SampleTime=2e-08
  rd_2 : Delay  DelayLength=double(6)  InitialCondition=0  InputProcessing=Inherited  SampleTime=2e-08
  rd_4 : Delay  DelayLength=double(2)  InitialCondition=0  InputProcessing=Inherited  SampleTime=2e-08
  rd_8 : Delay  DelayLength=double(5)  InitialCondition=0  InputProcessing=Inherited  SampleTime=2e-08
  reset_old{1..5} (5 alike) : Delay  DelayLength=double(1)  InitialCondition=0  InputProcessing=Inherited  SampleTime=2e-08
  reset_old_switch1 : Switch  Criteria=u2 ~= 0  Threshold=double(0)  OutDataTypeStr=uint16  SampleTime=2e-08
  reset_old_switch3 : Switch  Criteria=u2 ~= 0  Threshold=double(0)  OutDataTypeStr=boolean  SampleTime=2e-08
  omega : Outport
  omega_AXI4 : Outport  Port=2
  theta_el : Outport  Port=3
  theta_el_AXI4 : Outport  Port=4
  theta_mech_AXI4 : Outport  Port=5
  edge : Outport  Port=6
  count : Outport  Port=7
  direction_AXI4 : Outport  Port=8
  countPerPeriod_AXI4 : Outport  Port=9
  wires:
  ctr_0_1/1 -> Serializer_Subnetwork/2(in1), Serializer_Subnetwork1/2(in1)
  Product_theta_el/1 -> Product_theta_el0_deserializer/1(in0)
  Product_theta_el0_deserializer/1(out0) -> demux/1
  Serializer_Subnetwork1/1(out0) -> Product_theta_el/2
  mux1/1 -> Serializer_Subnetwork1/1(in0)
  Serializer_Subnetwork/1(out0) -> Product_theta_el/1
  mux/1 -> Serializer_Subnetwork/1(in0)
  out_8_pipe/1 -> delayMatch10/1
  delayMatch10/1 -> delayMatch9/1
  Constant1/1 -> reset_old_switch3/3
  reset_old_switch3/1 -> out_5_pipe/1
  Detec_edge/1 -> reset_old_switch1/2, reset_old_switch3/2
  reset_old_switch1/1 -> reset_old1/1
  Data Type Conversion9/1 -> Detec_edge/1, reset_old_switch1/1, reset_old5/1
  reset_old5/1 -> mux1/2
  demux/2 -> Product_theta_mech_out_dtc/1
  demux/1 -> Product_theta_el_out_dtc/1
  delayMatch8/1 -> mux/2
  reset_old2/1 -> mux1/1
  Data Type Conversion1/1 -> reset_old2/1
  delayMatch7/1 -> mux/1
  Product_theta_mech_out_dtc/1 -> reset_old3/1
  reset_old3/1 -> out_4_pipe/1
  out_4_pipe/1 -> delayMatch6/1
  Product_theta_el_out_dtc/1 -> reset_old4/1
  reset_old4/1 -> out_2_pipe/1, out_3_pipe/1
  out_2_pipe/1 -> delayMatch5/1
  out_3_pipe/1 -> delayMatch4/1
  reset_old1/1 -> Detec_edge/2, reset_old_switch1/3
  out_5_pipe/1 -> delayMatch3/1
  delayMatch3/1 -> delayMatch2/1
  Logical1_out_pipe/1 -> Counter/1(Enable_ctr), out_6_pipe/1
  Logical1/1 -> Logical1_out_pipe/1
  out_6_pipe/1 -> delayMatch1/1
  delayMatch1/1 -> delayMatch/1
  rd_11/1 -> Average/1("OmegaIn ")
  Data Type Conversion2/1 -> rd_11/1
  Average/1(OmegaOut) -> Mul_Direction/1, rd_10/1
  omega_by_measure_time/2(NewMeasurement) -> Average/2(NewMeasurement)
  omega_by_measure_time/1(rps) -> Mul_rps_omega/1
  Mul_rps_omega/1 -> Mul_rps_omega_out_dtc/1
  rd_9/1 -> Mul_Direction_out_dtc/1
  Mul_Direction/1 -> rd_9/1
  Mul_Direction_out_dtc/1 -> rd_8/1
  rd_7/1 -> Average/4(SamplingFactor)
  rd_6/1 -> Average/3(SamplingFactorInv)
  rd_5/1 -> omega_by_measure_time/2(T)
  rd_4/1 -> omega_by_measure_time/1(Edge)
  rd_3/1 -> Mul_rps_omega/2
  rd_1/1 -> Mul_Direction/2, rd_2/1
  Inc_PerTurn_mech_2PI_AXI4/1 -> delayMatch8/1
  PI2_Inc_AXI4/1 -> delayMatch7/1
  rd_0/1 -> rd_1/1, Counter_theta/4(Dir), Counter_theta_ele/4(Dir)
  Logical2/1 -> rd_4/1
  delayMatch9/1 -> countPerPeriod_AXI4/1
  rd_2/1 -> direction_AXI4/1
  delayMatch/1 -> count/1
  delayMatch2/1 -> edge/1
  delayMatch6/1 -> theta_mech_AXI4/1
  delayMatch4/1 -> theta_el_AXI4/1
  delayMatch5/1 -> theta_el/1
  rd_10/1 -> omega_AXI4/1
  rd_8/1 -> omega/1
  omega_by_count_lines/1(count) -> out_8_pipe/1
  Mul_rps_omega_out_dtc/1 -> HDL Reciprocal/1(In1)
  HDL Reciprocal/1(Out1) -> Data Type Conversion2/1
  Counter_theta_ele/1(count) -> Data Type Conversion1/1
  Counter_theta/1(count) -> Data Type Conversion9/1
  Counter/2(Reset) -> Counter_theta/2(Reset), Counter_theta_ele/2(Reset)
  Counter/1(Edge) -> Counter_theta/1(Edge), Counter_theta_ele/1(Edge), omega_by_count_lines/1(Edge)
  Constant/1 -> reset_old_switch3/1
  Check_Direction/1(Dir) -> rd_0/1
  C_1/rps->1/omega/1 -> rd_3/1
  PeriodEnd/1 -> omega_by_count_lines/2(Reset1)
  OverSamplFactor_AXI4/1 -> rd_7/1
  OverSamplFactorInv_AXI4/1 -> rd_6/1
  IncrementePerTurn_elek_AXI4/1 -> Counter_theta_ele/3(IncsPerTurn)
  IncPerTurn_mech_AXI4/1 -> Counter_theta/3(IncsPerTurn), omega_by_count_lines/3(IncsPerTurn)
  Timer_FPGA_ms_AXI4/1 -> rd_5/1
  I/1 -> Counter/2(I_line)
  B/1 -> Logical1/2, Check_Direction/2(B)
  A/1 -> Logical1/1, Check_Direction/1(A), Logical2/1

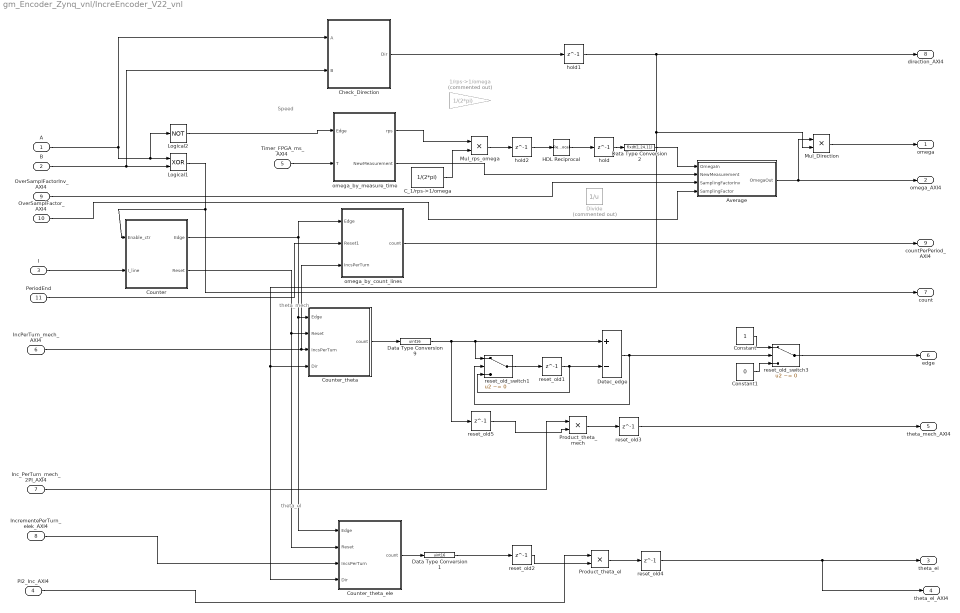
== system gm_Encoder_Zynq_vnl/IncreEncoder_V22_vnl ==
  note: theta_el
  note: theta_mech
  note: Speed
  A : Inport
  B : Inport  Port=2
  I : Inport  Port=3
  PI2_Inc_AXI4 : Inport  Port=4
  Timer_FPGA_ms_AXI4 : Inport  Port=5
  IncPerTurn_mech_AXI4 : Inport  Port=6
  Inc_PerTurn_mech_2PI_AXI4 : Inport  Port=7
  IncrementePerTurn_elek_AXI4 : Inport  Port=8
  OverSamplFactorInv_AXI4 : Inport  Port=9
  OverSamplFactor_AXI4 : Inport  Port=10
  PeriodEnd : Inport  Port=11
  1/rps->1/omega : Gain  Commented=on  Gain=1/(2*pi)  OutDataTypeStr=fixdt(1,24,18)
  Average : Subsystem
  C_1/rps->1/omega : Constant  Value=1/(2*pi)  OutDataTypeStr=fixdt(0,16,15)  SampleTime=-1
  Check_Direction : Subsystem  TreatAsAtomicUnit=on
  Constant : Constant  OutDataTypeStr=boolean  SampleTime=-1
  Constant1 : Constant  Value=0  OutDataTypeStr=boolean  SampleTime=-1
  Counter : Subsystem  TreatAsAtomicUnit=on
  Counter_theta : Subsystem  TreatAsAtomicUnit=on
  Counter_theta_ele : Subsystem  TreatAsAtomicUnit=on
  Data Type Conversion1 : DataTypeConversion  OutDataTypeStr=uint16
  Data Type Conversion2 : DataTypeConversion  OutDataTypeStr=fixdt(1,24,11)
  Data Type Conversion9 : DataTypeConversion  OutDataTypeStr=uint16
  Detec_edge : Sum  Inputs=+-  AccumDataTypeStr=uint8  OutDataTypeStr=uint8
  Divide : Math  Commented=on  Operator=reciprocal  OutDataTypeStr=fixdt(1,24,11)  RndMeth=Zero  SaturateOnIntegerOverflow=on
  HDL Reciprocal : Reciprocal
  Logical1 : Logic  Operator=XOR  AllPortsSameDT=off  OutDataTypeStr=boolean
  Logical2 : Logic  Operator=NOT  AllPortsSameDT=off  OutDataTypeStr=boolean
  Mul_Direction : Product  Inputs=**  SaturateOnIntegerOverflow=on  RndMeth=Zero  OutDataTypeStr=Inherit: Same as first input
  Mul_rps_omega : Product  Inputs=**  SaturateOnIntegerOverflow=on  RndMeth=Zero  OutDataTypeStr=Inherit: Same as first input
  Product_theta_el : Product  OutDataTypeStr=fixdt(1,24,20)
  Product_theta_mech : Product  OutDataTypeStr=fixdt(1,24,20)
  hold : Delay  DelayLength=1
  hold1 : Delay  DelayLength=1
  hold2 : Delay  DelayLength=1
  omega_by_count_lines : Subsystem  TreatAsAtomicUnit=on
  omega_by_measure_time : Subsystem  TreatAsAtomicUnit=on
  reset_old{1..5} (5 alike) : Delay  DelayLength=1
  reset_old_switch1 : Switch  Criteria=u2 ~= 0
  reset_old_switch3 : Switch  Criteria=u2 ~= 0
  omega : Outport
  omega_AXI4 : Outport  Port=2
  theta_el : Outport  Port=3
  theta_el_AXI4 : Outport  Port=4
  theta_mech_AXI4 : Outport  Port=5
  edge : Outport  Port=6
  count : Outport  Port=7
  direction_AXI4 : Outport  Port=8
  countPerPeriod_AXI4 : Outport  Port=9
  wires:
  omega_by_count_lines/1(count) -> countPerPeriod_AXI4/1
  PeriodEnd/1 -> omega_by_count_lines/2(Reset1)
  Data Type Conversion2/1 -> Average/1("OmegaIn ")
  Average/1(OmegaOut) -> Mul_Direction/1, omega_AXI4/1
  OverSamplFactor_AXI4/1 -> Average/4(SamplingFactor)
  omega_by_measure_time/2(NewMeasurement) -> Average/2(NewMeasurement)
  OverSamplFactorInv_AXI4/1 -> Average/3(SamplingFactorInv)
  Check_Direction/1(Dir) -> hold1/1
  hold2/1 -> HDL Reciprocal/1
  C_1/rps->1/omega/1 -> Mul_rps_omega/2
  Counter/1(Edge) -> Counter_theta/1(Edge), Counter_theta_ele/1(Edge), omega_by_count_lines/1(Edge)
  Counter/2(Reset) -> Counter_theta/2(Reset), Counter_theta_ele/2(Reset)
  Mul_Direction/1 -> omega/1
  Mul_rps_omega/1 -> hold2/1
  HDL Reciprocal/1 -> hold/1
  Timer_FPGA_ms_AXI4/1 -> omega_by_measure_time/2(T)
  Logical2/1 -> omega_by_measure_time/1(Edge)
  reset_old5/1 -> Product_theta_mech/2
  reset_old2/1 -> Product_theta_el/2
  Data Type Conversion1/1 -> reset_old2/1
  reset_old4/1 -> theta_el/1, theta_el_AXI4/1
  Counter_theta_ele/1(count) -> Data Type Conversion1/1
  PI2_Inc_AXI4/1 -> Product_theta_el/1
  IncrementePerTurn_elek_AXI4/1 -> Counter_theta_ele/3(IncsPerTurn)
  Data Type Conversion9/1 -> reset_old_switch1/1, Detec_edge/1, reset_old5/1
  omega_by_measure_time/1(rps) -> Mul_rps_omega/1
  IncPerTurn_mech_AXI4/1 -> Counter_theta/3(IncsPerTurn), omega_by_count_lines/3(IncsPerTurn)
  Logical1/1 -> Counter/1(Enable_ctr), count/1
  Detec_edge/1 -> reset_old_switch1/2, reset_old_switch3/2
  Constant1/1 -> reset_old_switch3/3
  reset_old_switch3/1 -> edge/1
  Constant/1 -> reset_old_switch3/1
  Product_theta_el/1 -> reset_old4/1
  Inc_PerTurn_mech_2PI_AXI4/1 -> Product_theta_mech/1
  Product_theta_mech/1 -> reset_old3/1
  reset_old3/1 -> theta_mech_AXI4/1
  reset_old1/1 -> Detec_edge/2, reset_old_switch1/3
  reset_old_switch1/1 -> reset_old1/1
  Counter_theta/1(count) -> Data Type Conversion9/1
  hold1/1 -> direction_AXI4/1, Counter_theta/4(Dir), Counter_theta_ele/4(Dir), Mul_Direction/2
  hold/1 -> Data Type Conversion2/1
  I/1 -> Counter/2(I_line)
  B/1 -> Logical1/2, Check_Direction/2(B)
  A/1 -> Logical1/1, Logical2/1, Check_Direction/1(A)

== system gm_Encoder_Zynq_vnl/IncrementalEncoder_Floating ==
  A : Inport
  B : Inport  Port=2
  I : Inport  Port=3
  poles : Inport  Port=4
  Add : Sum  Inputs=+-  OutDataTypeStr=fixdt(1,16,0)
  Counter3 : dspswit3/Counter  Direction=Up  CountEvent=Either edge  CounterSize=User defined  MaxCount=IncPerTurn*4  InitialCount=0  Output=Count  HitValue=32  ResetInput=on  SamplesPerFrame=1  Ts=1  CntDtype=double  HitDtype=Logical
  CutTheta_0_2PI : Subsystem
  Edge Detector2 : powerlib_meascontrol/Logic/Edge Detector  model=Rising  ic=0  Ts=-1
      settings: SourceProductName=Simscape Power Systems  SourceProductBaseCode=PS
  Edge Detector3 : powerlib_meascontrol/Logic/Edge Detector  model=Rising  ic=0  Ts=-1
      settings: SourceProductName=Simscape Power Systems  SourceProductBaseCode=PS
  Logical Operator1 : Logic  Operator=XOR  AllPortsSameDT=off  OutDataTypeStr=boolean
  Logical Operator3 : Logic  AllPortsSameDT=off  OutDataTypeStr=boolean
  Logical Operator4 : Logic  Operator=NOT  AllPortsSameDT=off  OutDataTypeStr=boolean
  Logical Operator5 : Logic  AllPortsSameDT=off  OutDataTypeStr=boolean
  Logical Operator6 : Logic  Operator=NOT  AllPortsSameDT=off  OutDataTypeStr=boolean
  Product : Product
  S-R Flip-Flop1 : simulink_extras/Flip Flops/S-R Flip-Flop  initial_condition=0
  Scope1 : Scope  NumInputPorts=4
  cut_theta_2pi : Gain  Gain=(2*pi)/IncPerTurn
  cut_theta_2pi1 : Gain  Gain=(2*pi)/IncPerTurn
  n_aus_theta_v4 : Subsystem
  rpm : Outport
  theta_mech : Outport  Port=2
  theta_elec : Outport  Port=3
  direction : Outport  Port=4
  wires:
  I/1 -> Counter3/2
  Counter3/1 -> cut_theta_2pi/1, Product/1, Scope1/1
  n_aus_theta_v4/1(n) -> rpm/1
  Logical Operator1/1 -> Scope1/4, Counter3/1
  cut_theta_2pi/1 -> Scope1/2, n_aus_theta_v4/1(theta), theta_mech/1
  Product/1 -> cut_theta_2pi1/1
  poles/1 -> Product/2
  cut_theta_2pi1/1 -> CutTheta_0_2PI/1(In1)
  CutTheta_0_2PI/1(Out1) -> theta_elec/1
  Edge Detector2/1 -> Logical Operator3/1
  Logical Operator4/1 -> Logical Operator3/2
  Logical Operator3/1 -> S-R Flip-Flop1/1
  Edge Detector3/1 -> Logical Operator5/1
  Logical Operator6/1 -> Logical Operator5/2
  Logical Operator5/1 -> S-R Flip-Flop1/2
  S-R Flip-Flop1/1 -> Add/1
  S-R Flip-Flop1/2 -> Add/2
  A/1 -> Logical Operator6/1, Edge Detector2/1, Logical Operator1/1
  B/1 -> Edge Detector3/1, Logical Operator4/1, Logical Operator1/2
  Add/1 -> direction/1

== system gm_Encoder_Zynq_vnl/ToCoverifySink ==
  in1 : Inport
  in2 : Inport  Port=2
  in3 : Inport  Port=3
  in4 : Inport  Port=4
  in5 : Inport  Port=5
  in6 : Inport  Port=6
  in7 : Inport  Port=7
  in8 : Inport  Port=8
  in9 : Inport  Port=9
  out1 : Outport
  out2 : Outport  Port=2
  out3 : Outport  Port=3
  out4 : Outport  Port=4
  out5 : Outport  Port=5
  out6 : Outport  Port=6
  out7 : Outport  Port=7
  out8 : Outport  Port=8
  out9 : Outport  Port=9
  tag scope: out1=global, out2=global, out3=global, out4=global, out5=global, out6=global, out7=global, out8=global, out9=global
  wires:
  in1/1 -> out1/1, [out1]
  in2/1 -> out2/1, [out2]
  in3/1 -> out3/1, [out3]
  in4/1 -> out4/1, [out4]
  in5/1 -> out5/1, [out5]
  in6/1 -> out6/1, [out6]
  in7/1 -> out7/1, [out7]
  in8/1 -> out8/1, [out8]
  in9/1 -> out9/1, [out9]

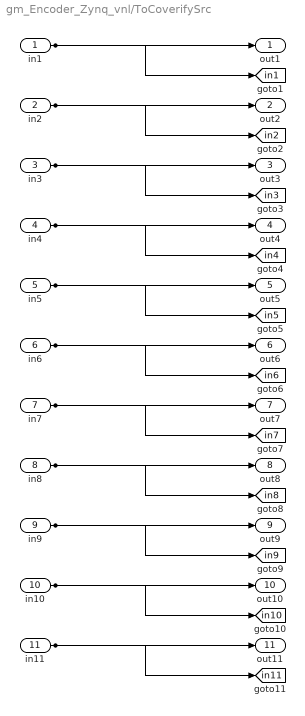
== system gm_Encoder_Zynq_vnl/ToCoverifySrc ==
  in1 : Inport
  in2 : Inport  Port=2
  in3 : Inport  Port=3
  in4 : Inport  Port=4
  in5 : Inport  Port=5
  in6 : Inport  Port=6
  in7 : Inport  Port=7
  in8 : Inport  Port=8
  in9 : Inport  Port=9
  in10 : Inport  Port=10
  in11 : Inport  Port=11
  out1 : Outport
  out2 : Outport  Port=2
  out3 : Outport  Port=3
  out4 : Outport  Port=4
  out5 : Outport  Port=5
  out6 : Outport  Port=6
  out7 : Outport  Port=7
  out8 : Outport  Port=8
  out9 : Outport  Port=9
  out10 : Outport  Port=10
  out11 : Outport  Port=11
  tag scope: in10=global, in11=global, in1=global, in2=global, in3=global, in4=global, in5=global, in6=global, in7=global, in8=global, in9=global
  wires:
  in1/1 -> out1/1, [in1]
  in2/1 -> out2/1, [in2]
  in3/1 -> out3/1, [in3]
  in4/1 -> out4/1, [in4]
  in5/1 -> out5/1, [in5]
  in6/1 -> out6/1, [in6]
  in7/1 -> out7/1, [in7]
  in8/1 -> out8/1, [in8]
  in9/1 -> out9/1, [in9]
  in10/1 -> out10/1, [in10]
  in11/1 -> out11/1, [in11]

== system gm_Encoder_Zynq_vnl/n_aus_theta ==
  count : Inport
  T : Inport  Port=2
  1/rps->1/omega : Gain  Gain=1/(2*pi)  OutDataTypeStr=double
  Add : Sum  Inputs=+-
  Add1 : Sum
  Constant : Constant  Value=0  OutDataTypeStr=double  SampleTime=-1
  Constant1 : Constant  Value=0  OutDataTypeStr=double  SampleTime=-1
  Constant2 : Constant  Value=0  OutDataTypeStr=double  SampleTime=-1
  Divide1 : Product  Inputs=/
  ProtectOverflow_T_count : Switch  Threshold=50
  ProtectOverflow_rps : Switch  Threshold=50  OutDataTypeStr=double
  Scope1 : Scope  NumInputPorts=4
  Scope2 : Scope  NumInputPorts=4
  T_count : Delay  DelayLength=1
  T_count_switch : Switch  Criteria=u2 ~= 0
  count_old : Delay  DelayLength=1
  count_old_switch : Switch  Criteria=u2 ~= 0
  speed_old : Delay  DelayLength=1
  speed_old_switch : Switch  Criteria=u2 ~= 0
  rpm : Outport
  wires:
  count_old_switch/1 -> count_old/1
  count_old/1 -> count_old_switch/3, Add/2
  Constant/1 -> T_count_switch/1
  Add/1 -> speed_old_switch/2, count_old_switch/2, Scope1/1, T_count_switch/2
  Constant1/1 -> ProtectOverflow_T_count/1
  ProtectOverflow_rps/1 -> 1/rps->1/omega/1, Scope2/1
  Constant2/1 -> ProtectOverflow_rps/1
  speed_old_switch/1 -> ProtectOverflow_rps/3, Scope2/3, speed_old/1
  speed_old/1 -> speed_old_switch/3
  T/1 -> Scope2/4, Add1/1
  ProtectOverflow_T_count/1 -> T_count/1
  T_count/1 -> Scope1/4, Add1/2
  Add1/1 -> Scope2/2, speed_old_switch/1, T_count_switch/3
  count/1 -> Add/1, count_old_switch/1
  T_count_switch/1 -> ProtectOverflow_rps/2, Scope1/2, ProtectOverflow_T_count/2, ProtectOverflow_T_count/3
  1/rps->1/omega/1 -> Divide1/1
  Divide1/1 -> rpm/1

== system gm_Encoder_Zynq_vnl/Compare/Assert_count ==
  cosim : Inport
  dut : Inport  Port=2
  AssertEq : Assertion  StopWhenAssertionFail=off
  Compare To Zero : simulink/Logic and Bit Operations/Compare To Zero  relop===  OutDataTypeStr=boolean
  Constant1 : Constant  Value=0  OutDataTypeStr=Inherit: Inherit via back propagation  SampleTime=-1
  Counter : simulink/Sources/Counter Free-Running  NumBits=32  tsamp=-1
  IgnoreCycles : Constant  Value=11  OutDataTypeStr=Inherit: Inherit via back propagation  SampleTime=-1
  Relational Operator : RelationalOperator  Operator=<  OutDataTypeStr=boolean  RndMeth=Nearest
  Relational Operator1 : RelationalOperator  Operator===  OutDataTypeStr=boolean  RndMeth=Nearest
  Switch : Switch  Criteria=u2 ~= 0
  Switch1 : Switch  Criteria=u2 ~= 0
  compare: count : Scope  NumInputPorts=3
  wires:
  Compare To Zero/1 -> compare: count/3
  Relational Operator1/1 -> Compare To Zero/1, AssertEq/1  "err"
  Switch1/1 -> compare: count/1, Relational Operator1/1
  Switch/1 -> compare: count/2, Relational Operator1/2
  Constant1/1 -> Switch/1, Switch1/1
  Relational Operator/1 -> Switch/2, Switch1/2
  cosim/1 -> Switch1/3  "cosim"
  dut/1 -> Switch/3  "dut ref"
  Counter/1 -> Relational Operator/1
  IgnoreCycles/1 -> Relational Operator/2

== system gm_Encoder_Zynq_vnl/Compare/Assert_countPerPeriod_AXI4 ==
  cosim : Inport
  dut : Inport  Port=2
  AssertEq : Assertion  StopWhenAssertionFail=off
  Compare To Zero : simulink/Logic and Bit Operations/Compare To Zero  relop===  OutDataTypeStr=boolean
  Constant1 : Constant  Value=0  OutDataTypeStr=Inherit: Inherit via back propagation  SampleTime=-1
  Counter : simulink/Sources/Counter Free-Running  NumBits=32  tsamp=-1
  IgnoreCycles : Constant  Value=11  OutDataTypeStr=Inherit: Inherit via back propagation  SampleTime=-1
  Relational Operator : RelationalOperator  Operator=<  OutDataTypeStr=boolean  RndMeth=Nearest
  Relational Operator1 : RelationalOperator  Operator===  OutDataTypeStr=boolean  RndMeth=Nearest
  Switch : Switch  Criteria=u2 ~= 0
  Switch1 : Switch  Criteria=u2 ~= 0
  compare: countPerPeriod_AXI4 : Scope  NumInputPorts=3
  wires:
  Compare To Zero/1 -> compare: countPerPeriod_AXI4/3
  Relational Operator1/1 -> Compare To Zero/1, AssertEq/1  "err"
  Switch1/1 -> compare: countPerPeriod_AXI4/1, Relational Operator1/1
  Switch/1 -> compare: countPerPeriod_AXI4/2, Relational Operator1/2
  Constant1/1 -> Switch/1, Switch1/1
  Relational Operator/1 -> Switch/2, Switch1/2
  cosim/1 -> Switch1/3  "cosim"
  dut/1 -> Switch/3  "dut ref"
  Counter/1 -> Relational Operator/1
  IgnoreCycles/1 -> Relational Operator/2

== system gm_Encoder_Zynq_vnl/Compare/Assert_direction_AXI4 ==
  cosim : Inport
  dut : Inport  Port=2
  AssertEq : Assertion  StopWhenAssertionFail=off
  Compare To Zero : simulink/Logic and Bit Operations/Compare To Zero  relop===  OutDataTypeStr=boolean
  Constant1 : Constant  Value=0  OutDataTypeStr=Inherit: Inherit via back propagation  SampleTime=-1
  Counter : simulink/Sources/Counter Free-Running  NumBits=32  tsamp=-1
  IgnoreCycles : Constant  Value=11  OutDataTypeStr=Inherit: Inherit via back propagation  SampleTime=-1
  Relational Operator : RelationalOperator  Operator=<  OutDataTypeStr=boolean  RndMeth=Nearest
  Relational Operator1 : RelationalOperator  Operator===  OutDataTypeStr=boolean  RndMeth=Nearest
  Switch : Switch  Criteria=u2 ~= 0
  Switch1 : Switch  Criteria=u2 ~= 0
  compare: direction_AXI4 : Scope  NumInputPorts=3
  wires:
  Compare To Zero/1 -> compare: direction_AXI4/3
  Relational Operator1/1 -> Compare To Zero/1, AssertEq/1  "err"
  Switch1/1 -> compare: direction_AXI4/1, Relational Operator1/1
  Switch/1 -> compare: direction_AXI4/2, Relational Operator1/2
  Constant1/1 -> Switch/1, Switch1/1
  Relational Operator/1 -> Switch/2, Switch1/2
  cosim/1 -> Switch1/3  "cosim"
  dut/1 -> Switch/3  "dut ref"
  Counter/1 -> Relational Operator/1
  IgnoreCycles/1 -> Relational Operator/2
